simulink model "MultiSensorsR2017b"  (R2018a)
settings: Solver=ode45  StartTime=0.0  StopTime=7  MaxStep=0.01  RelTol=1e-3  EnableMultiTasking=on
InitFcn:
  | WhiteNoise_Mean=0;
  | WhiteNoise_Variance=1;
  | 
  | WhiteNoise_Mean2=0;
  | WhiteNoise_Variance2=1;
  | 
  | F_amplitude = 1;
  | F_frequency =10; % rad/s
  | 
  | beta=10;
undefined symbols (not defined in the file): T_samp
settings Model: Creator=suki  LastModifiedBy=aksha
settings DataIOCC: LimitDataPoints=on  SaveFormat=Array
settings OptimizationCC: LifeSpan=inf
settings DebuggingCC: SolverPrmCheckMsg=warning  SFUnexpectedBacktrackingDiag=warning  SFNoUnconditionalDefaultTransitionDiag=warning  SFExecutionAtInitializationDiag=none
settings HardwareCC: ProdBitPerPointer=32  ProdBitPerSizeT=32  ProdBitPerPtrDiffT=32  ProdLargestAtomicFloat=None  ProdIntDivRoundTo=Undefined  ProdEndianess=Unspecified  ProdWordSize=32  ProdHWDeviceType=32-bit Generic
settings ModelReferenceCC: PropagateSignalLabelsOutOfModel=off
settings CodeAppCC: StateflowObjectComments=on
settings GRTTargetCC: TargetLangStandard=C89/C90 (ANSI)  GeneratePreprocessorConditionals=Disable all
settings ConfigComp: CovMetricSettings=dw  CovHtmlReporting=on  CovSaveCumulativeToWorkspaceVar=on  CovSaveSingleToWorkspaceVar=on  CovExternalEMLEnable=off  CovSFcnEnable=off

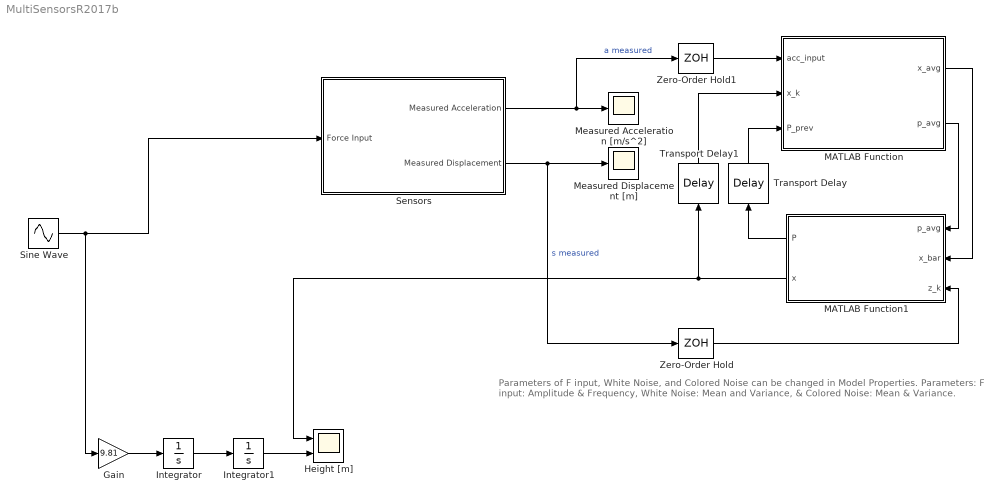
== system MultiSensorsR2017b ==
  note: Parameters of F input, White Noise, and Colored Noise can be changed in Model Properties.
      |
      | Parameters:
      | F input: Amplitude & Frequency,
      | White Noise: Mean and Variance, &
      | Colored Noise: Mean & Variance.
  Gain : Gain  Gain=9.81
  Height [m] : Scope  NumInputPorts=2
  Integrator : Integrator
  Integrator1 : Integrator
  MATLAB Function : MATLAB Function  TreatAsAtomicUnit=on
  MATLAB Function1 : MATLAB Function  TreatAsAtomicUnit=on
  Measured Acceleration [m/s^2] : Scope
  Measured Displacement [m] : Scope
  Sensors : Subsystem
  Sine Wave : Sin  Amplitude=F_amplitude  Frequency=F_frequency  Phase=6*rand  SampleTime=0
  Transport Delay : TransportDelay  DelayTime=T_samp  InitialOutput=[1 1 1; 1 1 1; 1 1 1]
  Transport Delay1 : TransportDelay  DelayTime=T_samp  InitialOutput=[0; 0; 0]
  Zero-Order Hold : ZeroOrderHold  SampleTime=T_samp
  Zero-Order Hold1 : ZeroOrderHold  SampleTime=T_samp
  wires:
  Sensors/1(Measured Acceleration) -> Measured Acceleration [m/s^2]/1, Zero-Order Hold1/1  "a measured"
  Sensors/2(Measured Displacement) -> Measured Displacement [m]/1, Zero-Order Hold/1  "s measured"
  MATLAB Function/2(p_avg) -> MATLAB Function1/1(p_avg)
  MATLAB Function1/1(P) -> Transport Delay/1
  MATLAB Function/1(x_avg) -> MATLAB Function1/2(x_bar)
  MATLAB Function1/2(x) -> Height [m]/1, Transport Delay1/1
  Zero-Order Hold1/1 -> MATLAB Function/1(acc_input)
  Zero-Order Hold/1 -> MATLAB Function1/3(z_k)
  Gain/1 -> Integrator/1
  Integrator1/1 -> Height [m]/2
  Sine Wave/1 -> Gain/1, Sensors/1(Force Input)
  Transport Delay/1 -> MATLAB Function/3(P_prev)
  Transport Delay1/1 -> MATLAB Function/2(x_k)
  Integrator/1 -> Integrator1/1

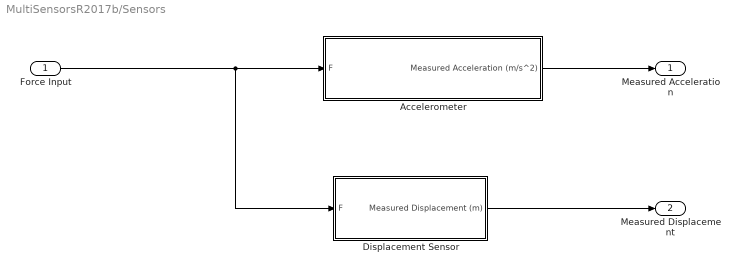
== system MultiSensorsR2017b/Sensors ==
  Force Input : Inport
  Accelerometer : Subsystem
  Displacement Sensor : Subsystem
  Measured Acceleration : Outport
  Measured Displacement : Outport  Port=2
  wires:
  Force Input/1 -> Accelerometer/1(F), Displacement Sensor/1(F)
  Displacement Sensor/1(Measured Displacement (m)) -> Measured Displacement/1
  Accelerometer/1(Measured Acceleration (m/s^2)) -> Measured Acceleration/1

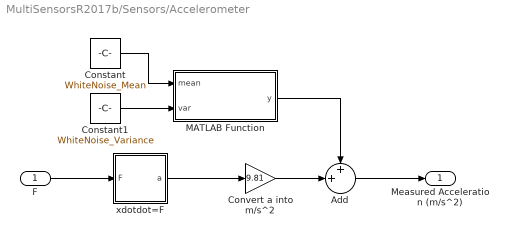
== system MultiSensorsR2017b/Sensors/Accelerometer ==
  F : Inport
  Add : Sum  Inputs=++|
  Constant : Constant  Value=WhiteNoise_Mean
  Constant1 : Constant  Value=WhiteNoise_Variance
  Convert a into m/s^2 : Gain  Gain=9.81
  MATLAB Function : MATLAB Function  TreatAsAtomicUnit=on
  xdotdot=F : Subsystem
  Measured Acceleration (m/s^2) : Outport
  wires:
  F/1 -> xdotdot=F/1(F)
  MATLAB Function/1(y) -> Add/1
  Convert a into m/s^2/1 -> Add/2
  xdotdot=F/1(a) -> Convert a into m/s^2/1
  Add/1 -> Measured Acceleration (m/s^2)/1
  Constant1/1 -> MATLAB Function/2(var)
  Constant/1 -> MATLAB Function/1(mean)

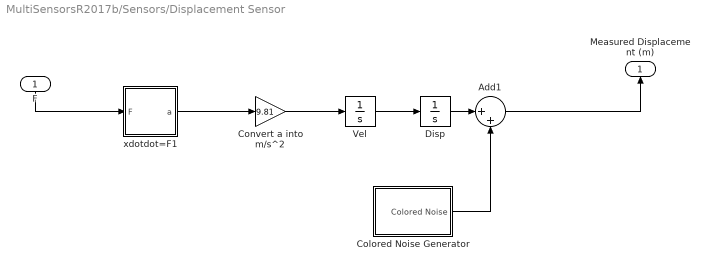
== system MultiSensorsR2017b/Sensors/Displacement Sensor ==
  F : Inport
  Add1 : Sum  Inputs=|++
  Colored Noise Generator : Subsystem
  Convert a into m/s^2 : Gain  Gain=9.81
  Disp : Integrator
  Vel : Integrator
  xdotdot=F1 : Subsystem
  Measured Displacement (m) : Outport
  wires:
  Colored Noise Generator/1(Colored Noise) -> Add1/2
  F/1 -> xdotdot=F1/1(F)
  Add1/1 -> Measured Displacement (m)/1
  Disp/1 -> Add1/1
  Vel/1 -> Disp/1
  xdotdot=F1/1(a) -> Convert a into m/s^2/1
  Convert a into m/s^2/1 -> Vel/1

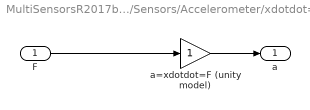
== system MultiSensorsR2017b/Sensors/Accelerometer/xdotdot=F ==
  F : Inport
  a=xdotdot=F (unity model) : Gain
  a : Outport
  wires:
  F/1 -> a=xdotdot=F (unity model)/1
  a=xdotdot=F (unity model)/1 -> a/1

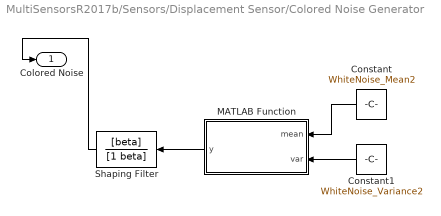
== system MultiSensorsR2017b/Sensors/Displacement Sensor/Colored Noise Generator ==
  Constant : Constant  Value=WhiteNoise_Mean2
  Constant1 : Constant  Value=WhiteNoise_Variance2
  MATLAB Function : MATLAB Function  TreatAsAtomicUnit=on
  Shaping Filter : TransferFcn  Numerator=[beta]  Denominator=[1 beta]
  Colored Noise : Outport
  wires:
  Shaping Filter/1 -> Colored Noise/1
  MATLAB Function/1(y) -> Shaping Filter/1
  Constant1/1 -> MATLAB Function/2(var)
  Constant/1 -> MATLAB Function/1(mean)

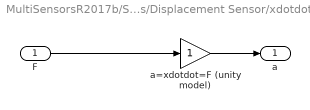
== system MultiSensorsR2017b/Sensors/Displacement Sensor/xdotdot=F1 ==
  F : Inport
  a=xdotdot=F (unity model) : Gain
  a : Outport
  wires:
  F/1 -> a=xdotdot=F (unity model)/1
  a=xdotdot=F (unity model)/1 -> a/1

== matlab function MultiSensorsR2017b/Sensors/Displacement Sensor/Colored Noise Generator/MATLAB Function ==
  data: mean input; y output; var input
function y = whitenoise(mean, var)

y = mean + sqrt(var)*randn;

== matlab function MultiSensorsR2017b/Sensors/Accelerometer/MATLAB Function ==
  data: mean input; y output; var input
function y = whitenoise(mean, var)

y = mean + sqrt(var)*randn;

== matlab function MultiSensorsR2017b/MATLAB Function ==
  data: acc_input input; x_k input; x_avg output; P_prev input; p_avg output
function [x_avg, p_avg] = TimeUpdateBox(acc_input, x_k, P_prev)

% The variance estimate of the acceleration and pressure sensor
var_acc = 1;
var_press = 1;
% The beta value given
beta = 100;
% The sampling time
T_samp = 0.01;

beta_v = -sqrt(2/beta)*var_press*(exp(-beta*T_samp)-1);

% Implementing Kalman Filter design
A = [1 T_samp 0; 0 1 0; 0 0 exp(-beta*T_samp)];
B = [0.5*T_samp*T_samp; T_samp; 0];
white_noise = [1 0 0; 0 1 0; 0 0 beta_v]*[var_acc var_acc var_press]';

Q = (B*B')*(white_noise*white_noise')*var_acc^2;

x_avg = A*x_k + B*acc_input;
p_avg = A*P_prev*(A') + Q;

== matlab function MultiSensorsR2017b/MATLAB Function1 ==
  data: p_avg input; x_bar input; z_k input; P output; x output
function [P, x] = MeasurementUpdateBox(p_avg, x_bar, z_k)

%The variance of the accelerometer
var_acc = 1; 

% The Kalman design for the measurement update section of the Kalman filter
C = [1 0 1];
R = var_acc*var_acc;

K = p_avg*C'*inv(C*p_avg*C' + R);
P = (eye(3) - K*C)*p_avg;
x = x_bar + K*(z_k - C*x_bar)';
